simulink model "TST_CoEng_StEng"  (R2016b)
settings: Solver=FixedStepDiscrete  StartTime=0.0  StopTime=simTime  FixedStep=sampleTime  RelTol=1e-3
values from neighbouring files (symbols this model uses):
  testCase = 1    [initTST_CoEng_StEng_001.m]    (also in initTST_CoEng_StEng_002.m = 2; initTST_CoEng_StEng_003.m = 3; initTST_CoEng_StEng_004.m = 4; initTST_CoEng_StEng_005.m = 5)
libraries: simulink x41, UnitTest_Lib x25
(part 2 of 2)

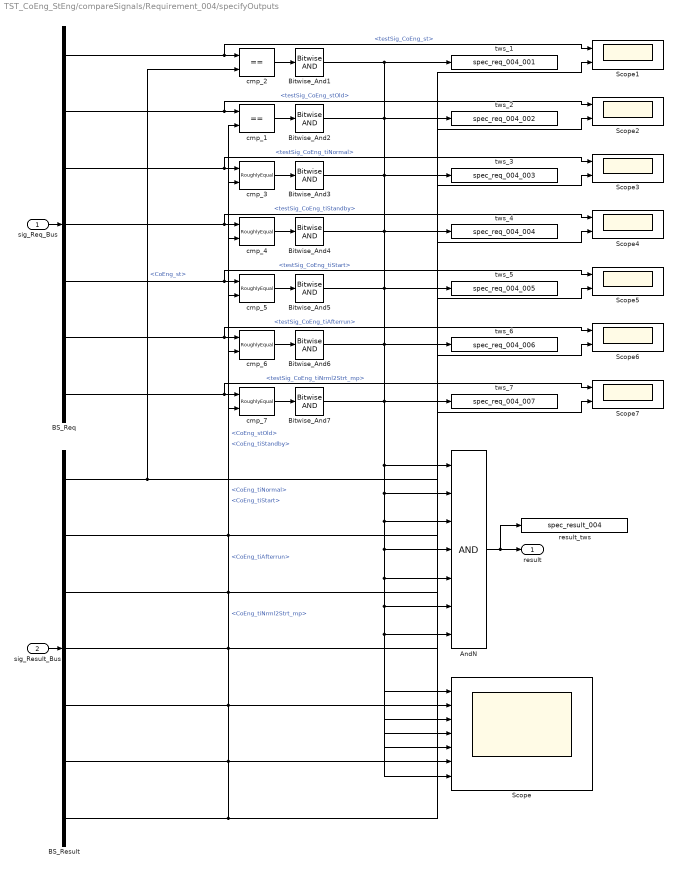
== system TST_CoEng_StEng/compareSignals/Requirement_004/specifyOutputs ==
  sig_Req_Bus : Inport
  sig_Result_Bus : Inport  Port=2
  AndN : Logic  Inputs=7
  BS_Req : BusSelector  OutputSignals=testSig_CoEng_st,testSig_CoEng_stOld,testSig_CoEng_tiNormal,testSig_CoEng_tiStandby,testSig_CoEng_tiStart,testSig_CoEng_tiAfterrun,testSig_CoEng_tiNrml2Strt_mp
  BS_Result : BusSelector  OutputSignals=CoEng_st,CoEng_stOld,CoEng_tiNormal,CoEng_tiStandby,CoEng_tiStart,CoEng_tiAfterrun,CoEng_tiNrml2Strt_mp
  Bitwise_And{1..7} (7 alike) : simulink/Logic and Bit Operations/Bitwise Operator  logicop=AND  UseBitMask=off  BitMask=bin2dec('11011001')  BitMaskRealWorld=Stored Integer
  Scope : Scope  NumInputPorts=7
  Scope{1..7} (7 alike) : Scope  NumInputPorts=2
  cmp_1 : RelationalOperator  Operator===  RndMeth=Nearest  InputSameDT=on
  cmp_2 : RelationalOperator  Operator===  RndMeth=Nearest  InputSameDT=on
  cmp_{3..7} (5 alike) : UnitTest_Lib/RoughlyEqual  slope=0.1
  result_tws : ToWorkspace  VariableName=spec_result_004
  tws_1 : ToWorkspace  VariableName=spec_req_004_001
  tws_2 : ToWorkspace  VariableName=spec_req_004_002
  tws_3 : ToWorkspace  VariableName=spec_req_004_003
  tws_4 : ToWorkspace  VariableName=spec_req_004_004
  tws_5 : ToWorkspace  VariableName=spec_req_004_005
  tws_6 : ToWorkspace  VariableName=spec_req_004_006
  tws_7 : ToWorkspace  VariableName=spec_req_004_007
  result : Outport
  wires:
  sig_Req_Bus/1 -> BS_Req/1
  sig_Result_Bus/1 -> BS_Result/1
  AndN/1 -> result/1, result_tws/1
  BS_Req/1 -> cmp_2/1, Scope1/1  "<testSig_CoEng_st>"
  BS_Result/1 -> cmp_2/2, Scope1/2  "<CoEng_st>"
  cmp_2/1 -> Bitwise_And1/1
  Bitwise_And1/1 -> AndN/1, Scope/1, tws_1/1
  BS_Req/2 -> cmp_1/1, Scope2/1  "<testSig_CoEng_stOld>"
  BS_Result/2 -> cmp_1/2, Scope2/2  "<CoEng_stOld>"
  cmp_1/1 -> Bitwise_And2/1
  Bitwise_And2/1 -> AndN/2, Scope/2, tws_2/1
  BS_Req/3 -> cmp_3/1, Scope3/1  "<testSig_CoEng_tiNormal>"
  BS_Result/3 -> cmp_3/2, Scope3/2  "<CoEng_tiNormal>"
  cmp_3/1 -> Bitwise_And3/1
  Bitwise_And3/1 -> AndN/3, Scope/3, tws_3/1
  BS_Req/4 -> cmp_4/1, Scope4/1  "<testSig_CoEng_tiStandby>"
  BS_Result/4 -> cmp_4/2, Scope4/2  "<CoEng_tiStandby>"
  cmp_4/1 -> Bitwise_And4/1
  Bitwise_And4/1 -> AndN/4, Scope/4, tws_4/1
  BS_Req/5 -> cmp_5/1, Scope5/1  "<testSig_CoEng_tiStart>"
  BS_Result/5 -> cmp_5/2, Scope5/2  "<CoEng_tiStart>"
  cmp_5/1 -> Bitwise_And5/1
  Bitwise_And5/1 -> AndN/5, Scope/5, tws_5/1
  BS_Req/6 -> cmp_6/1, Scope6/1  "<testSig_CoEng_tiAfterrun>"
  BS_Result/6 -> cmp_6/2, Scope6/2  "<CoEng_tiAfterrun>"
  cmp_6/1 -> Bitwise_And6/1
  Bitwise_And6/1 -> AndN/6, Scope/6, tws_6/1
  BS_Req/7 -> cmp_7/1, Scope7/1  "<testSig_CoEng_tiNrml2Strt_mp>"
  BS_Result/7 -> cmp_7/2, Scope7/2  "<CoEng_tiNrml2Strt_mp>"
  cmp_7/1 -> Bitwise_And7/1
  Bitwise_And7/1 -> AndN/7, Scope/7, tws_7/1

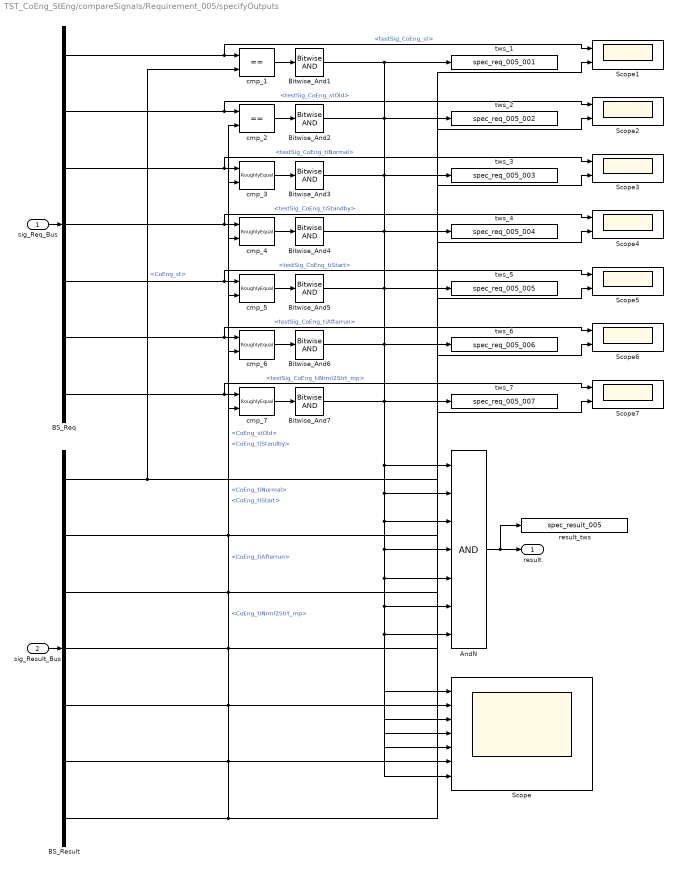
== system TST_CoEng_StEng/compareSignals/Requirement_005/specifyOutputs ==
  sig_Req_Bus : Inport
  sig_Result_Bus : Inport  Port=2
  AndN : Logic  Inputs=7
  BS_Req : BusSelector  OutputSignals=testSig_CoEng_st,testSig_CoEng_stOld,testSig_CoEng_tiNormal,testSig_CoEng_tiStandby,testSig_CoEng_tiStart,testSig_CoEng_tiAfterrun,testSig_CoEng_tiNrml2Strt_mp
  BS_Result : BusSelector  OutputSignals=CoEng_st,CoEng_stOld,CoEng_tiNormal,CoEng_tiStandby,CoEng_tiStart,CoEng_tiAfterrun,CoEng_tiNrml2Strt_mp
  Bitwise_And{1..7} (7 alike) : simulink/Logic and Bit Operations/Bitwise Operator  logicop=AND  UseBitMask=off  BitMask=bin2dec('11011001')  BitMaskRealWorld=Stored Integer
  Scope : Scope  NumInputPorts=7
  Scope{1..7} (7 alike) : Scope  NumInputPorts=2
  cmp_1 : RelationalOperator  Operator===  RndMeth=Nearest  InputSameDT=on
  cmp_2 : RelationalOperator  Operator===  RndMeth=Nearest  InputSameDT=on
  cmp_{3..7} (5 alike) : UnitTest_Lib/RoughlyEqual  slope=0.1
  result_tws : ToWorkspace  VariableName=spec_result_005
  tws_1 : ToWorkspace  VariableName=spec_req_005_001
  tws_2 : ToWorkspace  VariableName=spec_req_005_002
  tws_3 : ToWorkspace  VariableName=spec_req_005_003
  tws_4 : ToWorkspace  VariableName=spec_req_005_004
  tws_5 : ToWorkspace  VariableName=spec_req_005_005
  tws_6 : ToWorkspace  VariableName=spec_req_005_006
  tws_7 : ToWorkspace  VariableName=spec_req_005_007
  result : Outport
  wires:
  sig_Req_Bus/1 -> BS_Req/1
  sig_Result_Bus/1 -> BS_Result/1
  AndN/1 -> result/1, result_tws/1
  BS_Req/1 -> cmp_1/1, Scope1/1  "<testSig_CoEng_st>"
  BS_Result/1 -> cmp_1/2, Scope1/2  "<CoEng_st>"
  cmp_1/1 -> Bitwise_And1/1
  Bitwise_And1/1 -> AndN/1, Scope/1, tws_1/1
  BS_Req/2 -> cmp_2/1, Scope2/1  "<testSig_CoEng_stOld>"
  BS_Result/2 -> cmp_2/2, Scope2/2  "<CoEng_stOld>"
  cmp_2/1 -> Bitwise_And2/1
  Bitwise_And2/1 -> AndN/2, Scope/2, tws_2/1
  BS_Req/3 -> cmp_3/1, Scope3/1  "<testSig_CoEng_tiNormal>"
  BS_Result/3 -> cmp_3/2, Scope3/2  "<CoEng_tiNormal>"
  cmp_3/1 -> Bitwise_And3/1
  Bitwise_And3/1 -> AndN/3, Scope/3, tws_3/1
  BS_Req/4 -> cmp_4/1, Scope4/1  "<testSig_CoEng_tiStandby>"
  BS_Result/4 -> cmp_4/2, Scope4/2  "<CoEng_tiStandby>"
  cmp_4/1 -> Bitwise_And4/1
  Bitwise_And4/1 -> AndN/4, Scope/4, tws_4/1
  BS_Req/5 -> cmp_5/1, Scope5/1  "<testSig_CoEng_tiStart>"
  BS_Result/5 -> cmp_5/2, Scope5/2  "<CoEng_tiStart>"
  cmp_5/1 -> Bitwise_And5/1
  Bitwise_And5/1 -> AndN/5, Scope/5, tws_5/1
  BS_Req/6 -> cmp_6/1, Scope6/1  "<testSig_CoEng_tiAfterrun>"
  BS_Result/6 -> cmp_6/2, Scope6/2  "<CoEng_tiAfterrun>"
  cmp_6/1 -> Bitwise_And6/1
  Bitwise_And6/1 -> AndN/6, Scope/6, tws_6/1
  BS_Req/7 -> cmp_7/1, Scope7/1  "<testSig_CoEng_tiNrml2Strt_mp>"
  BS_Result/7 -> cmp_7/2, Scope7/2  "<CoEng_tiNrml2Strt_mp>"
  cmp_7/1 -> Bitwise_And7/1
  Bitwise_And7/1 -> AndN/7, Scope/7, tws_7/1
